simulink model "Trajectory_Teaching"  (R2016b)
settings: Solver=ode1  StartTime=0.0  StopTime=t_fin + 2*cut_time  FixedStep=T_sample  RelTol=1e-3  EnableMultiTasking=on
values from neighbouring files (symbols this model uses):
  cut_time = ceil(cut_time/T_sample_init)*T_sample_init    [Reference_Generation.m]
  t_fin = ceil(t_fin_init/T_sample_init)*T_sample_init    [Reference_Generation.m]
undefined symbols (not defined in the file or in its folder): Activator
libraries: simulink x2, qbmove_library x2, QB_pacer_lib x1
settings Model: Creator=Franco  LastModifiedBy=Franco
settings DataIOCC: LimitDataPoints=on  SaveFormat=Array
settings OptimizationCC: LifeSpan=inf
settings DebuggingCC: UnderspecifiedInitializationDetection=Classic  MergeDetectMultiDrivingBlocksExec=none  SolverPrmCheckMsg=warning  AllowSymbolicDim=off  StateNameClashWarn=warning  SFUnexpectedBacktrackingDiag=warning  SFNoUnconditionalDefaultTransitionDiag=warning  SFExecutionAtInitializationDiag=none
settings HardwareCC: ProdBitPerPointer=32  ProdBitPerSizeT=32  ProdBitPerPtrDiffT=32  ProdLargestAtomicFloat=None  ProdIntDivRoundTo=Undefined  ProdEndianess=Unspecified  ProdWordSize=32  ProdHWDeviceType=32-bit Generic
settings ModelReferenceCC: PropagateSignalLabelsOutOfModel=off
settings GRTTargetCC: TargetLangStandard=C89/C90 (ANSI)  GeneratePreprocessorConditionals=Disable all
settings ConfigComp: CovMetricSettings=dw  CovHtmlReporting=on  CovSaveCumulativeToWorkspaceVar=on  CovSaveSingleToWorkspaceVar=on  CovExternalEMLEnable=off  CovSFcnEnable=off

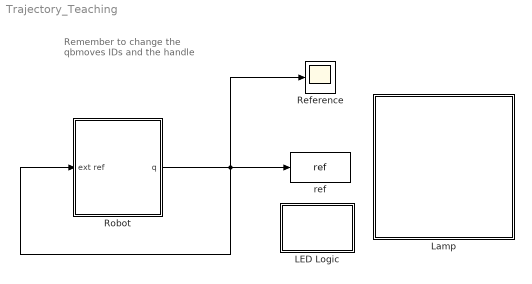
== system Trajectory_Teaching ==
  note: Remember to change the qbmoves IDs and the handle
  LED Logic : Subsystem
  Lamp : Subsystem  DialogController=hmiCreateDDGDialog  IsWebBlock=on  mask(MWDashboardBlock){webBlockId=f9ced507-b9df-4e29-8f0f-58b4c003cbd6, webBlockType=lamp, ShowInLibBrowser=on, ShowInitialText=on, HMISrcModelName=Trajectory_Teaching}
      mask prompts: webBlockType "WebBlock Type"; HMISrcModelName "Source Model"
      mask help: SimulinkHMI:dialogs:LampDialogDesc
      mask Help: helpview([docroot '/mapfiles/simulink.map'], 'hmi_lamp')
      mask Display:
      | if strcmp(get_param(bdroot(gcb),'BlockDiagramType'), 'library')
      |     image([(matlabroot) '/toolbox/simulink/hmi/icons/Lamp.png']);
      | end
  Reference : Scope
  Robot : Subsystem
  ref : ToWorkspace  VariableName=ref  SaveFormat=Timeseries  SampleTime=-1
  wires:
  Robot/1(q) -> Robot/1("ext ref "), Reference/1, ref/1

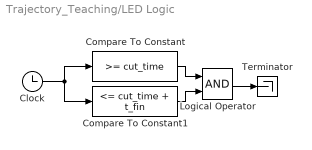
== system Trajectory_Teaching/LED Logic ==
  Clock : Clock
  Compare To Constant : simulink/Logic and Bit Operations/Compare To Constant  relop=>=  const=cut_time  OutDataTypeStr=boolean
  Compare To Constant1 : simulink/Logic and Bit Operations/Compare To Constant  relop=<=  const=cut_time + t_fin  OutDataTypeStr=boolean
  Logical Operator : Logic  AllPortsSameDT=off  OutDataTypeStr=boolean
  Terminator : Terminator
  wires:
  Compare To Constant1/1 -> Logical Operator/2
  Compare To Constant/1 -> Logical Operator/1
  Clock/1 -> Compare To Constant/1, Compare To Constant1/1
  Logical Operator/1 -> Terminator/1

== system Trajectory_Teaching/Lamp ==

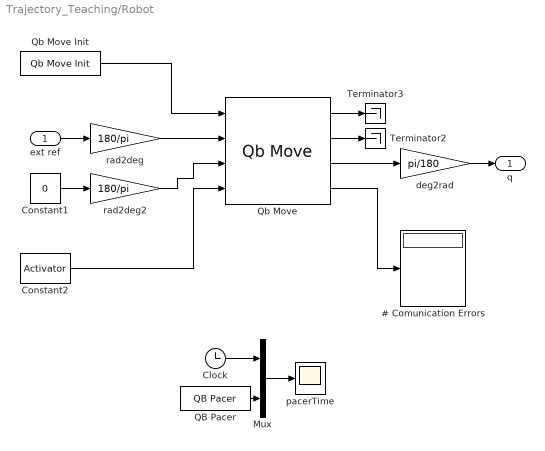
== system Trajectory_Teaching/Robot ==
  "ext ref " : Inport
  # Comunication Errors : Display
  Clock : Clock
  Constant1 : Constant  Value=0
  Constant2 : Constant  Value=Activator
  Mux : Mux  Inputs=2
  QB Pacer : QB_pacer_lib/QB Pacer  simTimePerRealTime=1
  Qb Move : qbmove_library/Qb Move  ID=[1 2 3 4 5 6]  ACTIVE_COMM_DIRECTIONS=Both  CONTROL_MODE=Equilibrium Position and Stiffness Preset  DAISY_CHAINING=off  MAX_ANG=0  SW_LIMIT=inf  OFFSET=0  ACTIVATE=off  WDT=0.0  UNIT=Degrees
  Qb Move Init : qbmove_library/Qb Move Init  NUMBER_OF_COM='COM7'  BAUD_RATE_COM=2000000
  Terminator2 : Terminator
  Terminator3 : Terminator
  deg2rad : Gain  Gain=pi/180
  pacerTime : Scope
  rad2deg : Gain  Gain=180/pi
  rad2deg2 : Gain  Gain=180/pi
  q : Outport
  wires:
  deg2rad/1 -> q/1
  "ext ref "/1 -> rad2deg/1
  Constant1/1 -> rad2deg2/1
  QB Pacer/1 -> Mux/2
  Clock/1 -> Mux/1
  Qb Move Init/1 -> Qb Move/1
  Mux/1 -> pacerTime/1
  Qb Move/1 -> Terminator3/1
  Qb Move/2 -> Terminator2/1
  Qb Move/3 -> deg2rad/1
  rad2deg/1 -> Qb Move/2
  Qb Move/4 -> # Comunication Errors/1
  rad2deg2/1 -> Qb Move/3
  Constant2/1 -> Qb Move/4
